simulink model "test_awls_estimators"  (R2024b)
settings: Solver=FixedStepDiscrete  StartTime=0.0  StopTime=0.5  FixedStep=Ts  RelTol=1e-3
model workspace (MAT data in the model file):
  Ts = Simulink.Parameter
  Ts.Value = 0.001
  Ts.Complexity = 'real'
  Ts.Dimensions = [1 1]
  Ts.Description = 'Sample time.'
  Ts.DataType = 'auto'
  Ts.DocUnits = 's'
libraries: dspsrcs4 x3, dspobslib x3, dspbuff3 x2, arsenal x2, dspswit3 x1
settings Model: Creator=Carchesion  LastModifiedBy=upattacini
settings SolverCC: AlgebraicLoopSolver=TrustRegion
settings DataIOCC: SaveFormat=Array  SignalLoggingSaveFormat=ModelDataLogs  SaveOutput=off  SignalLogging=off  SaveTime=off  ReturnWorkspaceOutputs=off
settings OptimizationCC: ExpressionDepthLimit=2147483647  InitFltsAndDblsToZero=on  LifeSpan=inf
settings DebuggingCC: UnderspecifiedInitializationDetection=Classic  MergeDetectMultiDrivingBlocksExec=none  SolverPrmCheckMsg=warning  FcnCallInpInsideContextMsg=warning  UnconnectedInputMsg=warning  UnconnectedOutputMsg=warning  UnconnectedLineMsg=warning  StateNameClashWarn=warning  SFUnexpectedBacktrackingDiag=warning  SFNoUnconditionalDefaultTransitionDiag=warning  SFExecutionAtInitializationDiag=none  ArithmeticOperatorsInVariantConditions=warning
settings HardwareCC: ProdBitPerPointer=32  ProdBitPerSizeT=32  ProdBitPerPtrDiffT=32  ProdLargestAtomicFloat=None  ProdIntDivRoundTo=Undefined  ProdEndianess=Unspecified  ProdWordSize=32  ProdHWDeviceType=32-bit Generic
settings ModelReferenceCC: EnableRefExpFcnMdlSchedulingChecks=on  PropagateSignalLabelsOutOfModel=off
settings SFSimCC: SimUseLocalCustomCode=off  SimParseCustomCode=off  CustomCodeUndefinedFunction=UseInterfaceOnly
settings RTWCC: RTWUseLocalCustomCode=off  GPUComputeCapability=3.5
settings CodeAppCC: StateflowObjectComments=on
settings GRTTargetCC: TargetLangStandard=C89/C90 (ANSI)  CombineOutputUpdateFcns=off  GRTInterface=on
settings ConfigComp: CovMetricSettings=dw  CovSaveCumulativeToWorkspaceVar=on  CovSaveSingleToWorkspaceVar=on  CovExternalEMLEnable=off

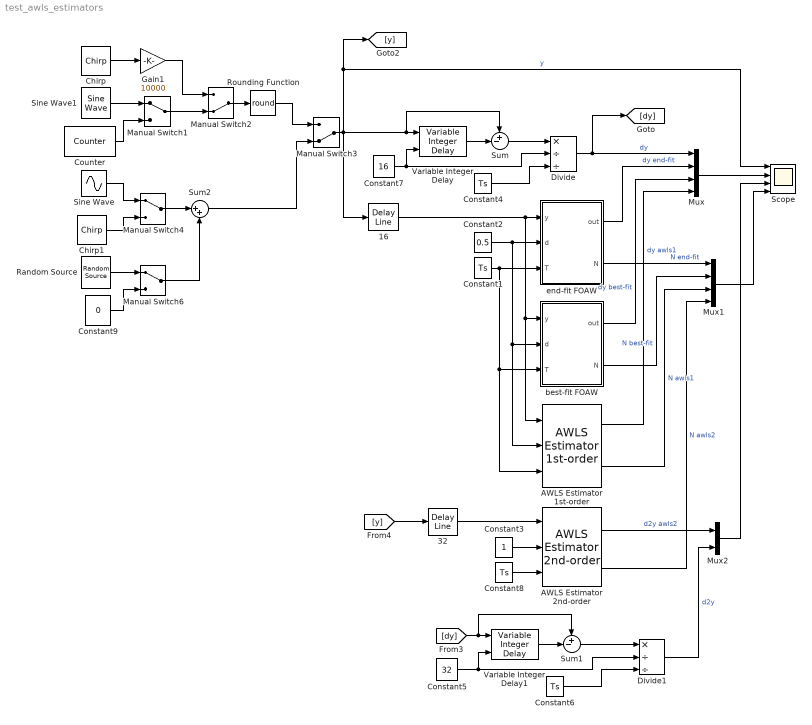
== system test_awls_estimators ==
  16 : dspbuff3/Delay Line  siz=16  ic=0  directfeed=off  enable_output=off  hold_output=off  OutputFrames=on
  32 : dspbuff3/Delay Line  siz=32  ic=0  directfeed=off  enable_output=off  hold_output=off  OutputFrames=on
  AWLS Estimator 1st-order : arsenal/Estimators/Adaptive Window Least-Squares Estimators/AWLS Estimator 1st-order  Description=This block implements adaptive window techniques as per https://dx.doi.org/10.1109/87.880606.  SystemSampleTime=-1  VariantActivationTime=update diagram  AllowFlexibleInterface=on  Latency=0  AutoFrameSizeCalculation=off
      settings: SourceProductName=iCub Tech Arsenal
  AWLS Estimator 2nd-order : arsenal/Estimators/Adaptive Window Least-Squares Estimators/AWLS Estimator 2nd-order  Description=This block implements adaptive window techniques as per https://dx.doi.org/10.1109/87.880606.  SystemSampleTime=-1  VariantActivationTime=update diagram  AllowFlexibleInterface=on  Latency=0  AutoFrameSizeCalculation=off
      settings: SourceProductName=iCub Tech Arsenal
  Chirp : dspsrcs4/Chirp  sweep=Linear  mode=Bidirectional  f0=0  f1=5  t1=1  Tsweep=1  phase=0  Ts=Ts  spf=1  datatype=double  OutputFrames=on
  Chirp1 : dspsrcs4/Chirp  sweep=Linear  mode=Bidirectional  f0=0  f1=10  t1=0.5  Tsweep=0.5  phase=0  Ts=Ts  spf=1  datatype=double  OutputFrames=on
  Constant{1,4,6,8} (4 alike) : Constant  Value=Ts
  Constant2 : Constant  Value=0.5
  Constant3 : Constant
  Constant5 : Constant  Value=32
  Constant7 : Constant  Value=16
  Constant9 : Constant  Value=0
  Counter : dspswit3/Counter  Direction=Up  CountEvent=Free running  CounterSize=32 bits  MaxCount=255  InitialCount=0  Output=Count  HitValue=32  ResetInput=off  SamplesPerFrame=1  Ts=Ts  CntDtype=double  HitDtype=Logical
  Divide : Product  Inputs=*//
  Divide1 : Product  Inputs=*//
  Gain1 : Gain  Gain=10000
  Manual Switch1 : ManualSwitch
  Manual Switch2 : ManualSwitch  CurrentSetting=0
  Manual Switch3 : ManualSwitch  CurrentSetting=0
  Manual Switch4 : ManualSwitch
  Manual Switch6 : ManualSwitch
  Mux : Mux
  Mux1 : Mux
  Mux2 : Mux  Inputs=2
  Random Source : dspobslib/Random Source  SrcType=Gaussian  NormMethod=Ziggurat  CltLength=12  MinVal=0  MaxVal=1  MeanVal=0  VarVal=1e-3  RepMode=Not repeatable  rawSeed=1  IsInherit=off  SampMode=Discrete  SampTime=Ts  SampFrame=1  DataType=Double  OutComplex=Real  OutputFrames=on
  Rounding Function : Rounding  Operator=round
  Scope : Scope  NumInputPorts=4
  Sine Wave : Sin  Frequency=2*pi*5  SampleTime=Ts
  Sine Wave1 : dspsrcs4/Sine Wave  Amplitude=10  Frequency=0.1  Phase=0  SampleMode=Discrete  OutComplex=Real  CompMethod=Trigonometric fcn  TableSize=Speed  SampleTime=Ts  SamplesPerFrame=1  ResetState=Restart at time zero  OutputFrames=on  dataType=double  wordLen=16  udDataType=sfix(16)  fracBitsMode=Best precision  numFracBits=15  OutDataTypeStr=double  LastOutDataTypeStr=double
  Sum : Sum  Inputs=+-|
  Sum1 : Sum  Inputs=+-|
  Sum2 : Sum  Inputs=|++
  Variable Integer Delay : dspobslib/Variable Integer Delay  dmax=1024  InputProcessing=Columns as channels (frame based)  ic=0  noDFT=off
  Variable Integer Delay1 : dspobslib/Variable Integer Delay  dmax=1024  InputProcessing=Columns as channels (frame based)  ic=0  noDFT=off
  best-fit FOAW : MATLAB Function  TreatAsAtomicUnit=on
  end-fit FOAW : MATLAB Function  TreatAsAtomicUnit=on
  wires:
  Counter/1 -> Manual Switch1/2
  Sine Wave1/1 -> Manual Switch1/1
  Constant1/1 -> end-fit FOAW/3(T), AWLS Estimator 1st-order/3, best-fit FOAW/3(T)
  Constant2/1 -> end-fit FOAW/2(d), AWLS Estimator 1st-order/2, best-fit FOAW/2(d)
  Mux/1 -> Scope/2
  end-fit FOAW/2(N) -> Mux1/1  "N end-fit"
  best-fit FOAW/2(N) -> Mux1/2  "N best-fit"
  best-fit FOAW/1(out) -> Mux/3  "dy best-fit"
  Manual Switch3/1 -> 16/1, Variable Integer Delay/1, Sum/1, Scope/1, [y]  "y"
  16/1 -> end-fit FOAW/1(y), AWLS Estimator 1st-order/1, best-fit FOAW/1(y)
  Manual Switch1/1 -> Manual Switch2/2
  Manual Switch2/1 -> Rounding Function/1
  Chirp/1 -> Gain1/1
  Gain1/1 -> Manual Switch2/1
  Variable Integer Delay/1 -> Sum/2
  Constant7/1 -> Variable Integer Delay/2, Divide/2
  Sum/1 -> Divide/1
  Divide/1 -> [dy], Mux/1  "dy"
  Constant4/1 -> Divide/3
  AWLS Estimator 1st-order/2 -> Mux1/3  "N awls1"
  AWLS Estimator 2nd-order/2 -> Mux1/4  "N awls2"
  Mux1/1 -> Scope/4
  [dy] -> Sum1/1, Variable Integer Delay1/1
  Variable Integer Delay1/1 -> Sum1/2
  Constant5/1 -> Variable Integer Delay1/2, Divide1/2
  Sum1/1 -> Divide1/1
  Constant6/1 -> Divide1/3
  Divide1/1 -> Mux2/2  "d2y"
  Mux2/1 -> Scope/3
  AWLS Estimator 2nd-order/1 -> Mux2/1  "d2y awls2"
  Constant3/1 -> AWLS Estimator 2nd-order/2
  32/1 -> AWLS Estimator 2nd-order/1
  [y] -> 32/1
  Constant8/1 -> AWLS Estimator 2nd-order/3
  Rounding Function/1 -> Manual Switch3/1
  Sine Wave/1 -> Manual Switch4/1
  Manual Switch4/1 -> Sum2/1
  Random Source/1 -> Manual Switch6/1
  Constant9/1 -> Manual Switch6/2
  Manual Switch6/1 -> Sum2/2
  Chirp1/1 -> Manual Switch4/2
  Sum2/1 -> Manual Switch3/2
  AWLS Estimator 1st-order/1 -> Mux/4  "dy awls1"
  end-fit FOAW/1(out) -> Mux/2  "dy end-fit"

== matlab function test_awls_estimators/best-fit FOAW ==
  data: y input; out output; d input; T input; N output
function [out,N]=fcn(y,d,T)

L=length(y);
bn=0;

for N=1:L-1
    an=y(L-N);
    bn=0;
    for i=0:N
        bn=bn+(N-2*i)*y(L-i);
    end
    bn=bn/(T*N*(N+1)*(N+2)/6);
    
    finish=false;
    for i=1:N-1
        Ly=an+bn*(N-i)*T;
        if abs(y(L-i)-Ly)>d
            finish=true;
            break;
        end
    end
    
    if finish
        break;
    end
end

out=bn;

== matlab function test_awls_estimators/end-fit FOAW ==
  data: y input; out output; d input; T input; N output
function [out,N]=fcn(y,d,T)

L=length(y);
bn=0;

for N=1:L-1
    an=y(L-N);
    bn=(y(L)-y(L-N))/(N*T);

    finish=false;
    for i=1:N-1
        Ly=an+bn*(N-i)*T;
        if abs(y(L-i)-Ly)>d
            finish=true;
            break;
        end
    end
    
    if finish
        break;
    end
end

out=bn;
